simulink model "realimentacion_ee"  (R2021a)
settings: Solver=VariableStepAuto  StartTime=0.0  StopTime=10.0  RelTol=1e-3
values from neighbouring files (symbols this model uses):
  A = [-2 -1; 0 -4]    [Control_Integral.m]    (also in Controlabilidad.m = P.a; Ejemplo_filminas.m = SS.A; Ejercicio_Inestable.m = [100, 0; 160, 200]; Ejercicio_Valvulas.m = double(A))
  B = [1; 0]    [Control_Integral.m]    (also in Controlabilidad.m = P.b; Ejemplo_filminas.m = SS.B; Ejercicio_Inestable.m = [70; 160]; Ejercicio_Valvulas.m = double(B))
  C = [1 1]    [Control_Integral.m]    (also in Controlabilidad.m = P.c; Ejemplo_filminas.m = SS.C; Ejercicio_Inestable.m = [1, 1]; Ejercicio_Valvulas.m = double(C))
  K = [p1-a1 p2-a2] * Wrm * inv(Wr)    [Controlabilidad.m]    (also in Ejemplo_filminas.m; Ejercicio_Inestable.m = [p1 - a1, p2 - a2] * Wrm * inv(Wr); Ejercicio_Valvulas.m = Ka(1:order(P)); realimentacion_ee.m = acker(A, B, [-10 -10]))
  kf = -1/(C*inv(A - B*K) * B)    [Controlabilidad.m]    (also in Ejemplo_filminas.m = -1/(Ccl * inv(Acl)*Bcl); Ejercicio_Inestable.m = 1/(-(C - D*K) * inv(A - B*K) * B + D); realimentacion_ee.m = 10)
  L = zpk(ceros, polos, ganancia)    [Ejemplo_filminas.m]    (also in Ejercicio_Inestable.m = inv(Wo) * Wom * [l1 - a1; l2 - a2]; Observabilidad.m = [18; 99]; realimentacion_ee.m = [18; 99])
settings Model: Creator=Santiago  LastModifiedBy=Santiago

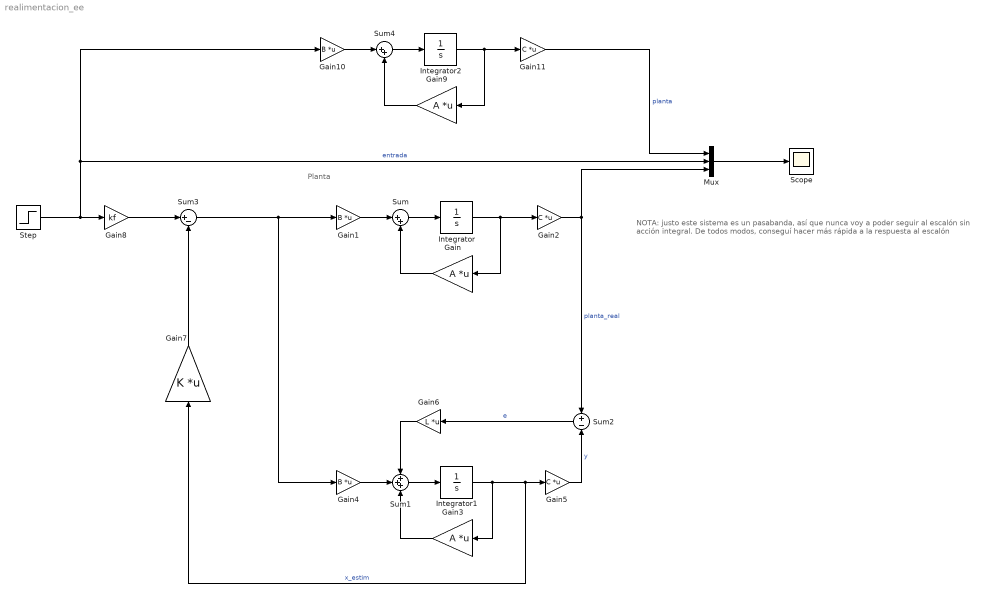
== system realimentacion_ee ==
  note: NOTA: justo este sistema es un pasabanda, así que nunca voy a poder
      | seguir al escalón sin acción integral. De todos modos, conseguí hacer más rápida a la respuesta al escalón
  note: Planta
  Gain : Gain  Gain=A  Multiplication=Matrix(K*u) (u vector)
  Gain1 : Gain  Gain=B  Multiplication=Matrix(K*u)
  Gain10 : Gain  Gain=B  Multiplication=Matrix(K*u)
  Gain11 : Gain  Gain=C  Multiplication=Matrix(K*u)
  Gain2 : Gain  Gain=C  Multiplication=Matrix(K*u)
  Gain3 : Gain  Gain=A  Multiplication=Matrix(K*u) (u vector)
  Gain4 : Gain  Gain=B  Multiplication=Matrix(K*u)
  Gain5 : Gain  Gain=C  Multiplication=Matrix(K*u)
  Gain6 : Gain  Gain=L  Multiplication=Matrix(K*u)
  Gain7 : Gain  Gain=K  Multiplication=Matrix(K*u) (u vector)
  Gain8 : Gain  Gain=kf
  Gain9 : Gain  Gain=A  Multiplication=Matrix(K*u) (u vector)
  Integrator : Integrator
  Integrator1 : Integrator
  Integrator2 : Integrator
  Mux : Mux  Inputs=3
  Scope : Scope
  Step : Step  SampleTime=0
  Sum : Sum  Inputs=|++
  Sum1 : Sum  Inputs=+++
  Sum2 : Sum  Inputs=+|-
  Sum3 : Sum  Inputs=|+-
  Sum4 : Sum  Inputs=|++
  wires:
  Gain1/1 -> Sum/1
  Gain/1 -> Sum/2
  Sum/1 -> Integrator/1
  Integrator/1 -> Gain2/1, Gain/1
  Sum1/1 -> Integrator1/1
  Gain4/1 -> Sum1/2
  Integrator1/1 -> Gain5/1, Gain7/1, Gain3/1  "x_estim"
  Gain3/1 -> Sum1/3
  Gain6/1 -> Sum1/1
  Sum2/1 -> Gain6/1  "e"
  Gain5/1 -> Sum2/2  "y"
  Gain2/1 -> Mux/3, Sum2/1  "planta_real"
  Step/1 -> Gain10/1, Mux/2, Gain8/1  "entrada"
  Gain8/1 -> Sum3/1
  Gain7/1 -> Sum3/2
  Sum3/1 -> Gain4/1, Gain1/1
  Sum4/1 -> Integrator2/1
  Gain10/1 -> Sum4/1
  Integrator2/1 -> Gain11/1, Gain9/1
  Gain9/1 -> Sum4/2
  Mux/1 -> Scope/1
  Gain11/1 -> Mux/1  "planta"
